simulink model "panda_test_1"  (Simulink 7.9)
settings: Solver=FixedStepDiscrete  StartTime=0.0  StopTime=inf  FixedStep=1  RelTol=1e-3
undefined symbols (not defined in the file): none, videoinput
libraries: imaqlib x1
settings Model: Creator=wildcat  LastModifiedBy=wildcat
settings RTWCC: SystemTargetFile=rlnx.tlc  GenCodeOnly=on  TemplateMakefile=rlnx_ubuntu.tmf  Description=Linux Real-Time Target  ProcessScript=rlnx_make_rtw_hook
settings CodeAppCC: GenerateComments=off  SimulinkBlockComments=off
settings STFCustomTargetCC: CodeReplacementLibrary=ANSI_C  ModelReferenceCompliant=off  GeneratePreprocessorConditionals=Disable all  MatFileLogging=on  SystemTargetFile=rlnx.tlc
settings GRTTargetCC: ModelReferenceCompliant=off  ParMdlRefBuildCompliant=off  CompOptLevelCompliant=off  ConcurrentExecutionCompliant=off  CombineOutputUpdateFcns=off  GRTInterface=on
settings CustomProperty: DataType=string  Value=-lm -ldl
settings EnumStrPairs: String=PC

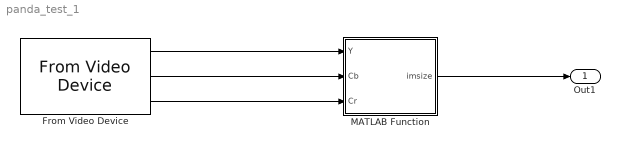
== system panda_test_1 ==
  From Video Device : imaqlib/From Video Device  DeviceMenu=winvideo 1 (Integrated Webcam)  Device=winvideo 1 (Microsoft LifeCam HD-3000)  ObjConstructor=videoinput('winvideo', 1)  VideoFormatMenu=YUY2_1280x720  VideoFormat=YUY2_1280x720  VideoSource=input1  ROIPosition=[0 0 720 1280]  EnableHWTrigger=off  TriggerConfiguration=none/none  SampleTime=1/30  OutputPortsMode=Separate color signals  DataType=uint8  CanDoHWTrigger=no  ReturnedColorSpace=YCbCr  BlockHandle=4.001  ROIWidth=1280  ROIHeight=720  ROIColumn=0  ROIRow=0  EngXMLPath=C:\Program Files\MATLAB\R2012a\toolbox\imaq\imaq\private  DevXMLPath=C:\Program Files\MATLAB\R2012a\toolbox\imaq\imaqadaptors\win64  EngLibPath=C:\Program Files\MATLAB\R2012a\toolbox\imaq\imaqblks\imaqmex\win64  ColorSpace=rgb  BayerSensorAlignment=grbg
  MATLAB Function : MATLAB Function  TreatAsAtomicUnit=on
  Out1 : Outport
  wires:
  From Video Device/1 -> MATLAB Function/1(Y)
  From Video Device/2 -> MATLAB Function/2(Cb)
  From Video Device/3 -> MATLAB Function/3(Cr)
  MATLAB Function/1(imsize) -> Out1/1

== matlab function MATLAB Function ==
  data: Y input double; imsize output double; Cb input double; Cr input double
function imsize = fcn(Y,Cb,Cr)
%#codegen

Y=uint32(Y);
Cb=uint32(Cb);
Cr=uint32(Cr);

size1=size(Y);
size2=size(Cb);
size3=size(Cr);

imsize=(size1+size2+size3)/3;
